simulink model "sim660"  (R2025a)
settings: Solver=ode23s  StartTime=0.0  StopTime=10000  RelTol=1e-3
model workspace (MAT data in the model file):
  op_snapshot1 : opcond.OperatingPoint (value not decoded)
undefined symbols (not defined in the file or in its folder): State132MW, State198MW, State198MW_DELAY
libraries: slpidlib x4, simulink x2, adrc_toolbox_library x1
(part 5 of 5)

== matlab function sim660/Subsystem/MATLAB Function2 ==
  data: pst input; hst input; Dst output; u input
function Dst= Dst(pst,hst,u)
%#codegen

%Dst=u*pst*(-0.0011*hst+4.399);
Dst=0.406*u*pst;
end

== matlab function sim660/MATLAB Function3 ==
  data: Td output; pm input; hm input
function Td = Td(pm, hm)
pm = pm;
hm = hm;
Td = T_ph(pm,hm)-273.15;
end



%% stand alone functions
function T = T_ph(p,h)
% T = T_ph(p,h)
%   Temperature of liquid, vapor or mixture, T [K], as functions of pressure, p [MPa], and enthalpy, h [kJ/kg]
% based on IAPWS-IF97
% Reference: http://www.iapws.org/
% June 2, 2009
% Mark Mikofski
%% size of inputs
dim = size(p);
initnan = NaN(dim);
T = initnan;
%% constants and calculated scalars
Tmin = 273.16; % [K] minimum temperature is triple point
T2bcsat = 554.485; % [K] saturation temperature at 5.85 kJ/kg/K isentropic line between region 2b and 2c
TB13 = 623.15; % [K] temperature at boundary between region 1 and 3
Tmax = 1073.15; % [K] maximum temperature
pmin = psat_T(Tmin); % [MPa] minimum pressure is 611.657 Pa
p2ab = 4; % [MPa] pressure along boundary between region 2a and 2b
p2bcsat = psat_T(T2bcsat); % [MPa] saturation pressure at 5.85 kJ/kg/K isentropic line between region 2b and 2c
pB13sat = psat_T(TB13); % [MPa] saturation pressure at boundary between region 1 and 3, 16.5291643 MPa
pmax = 100; % [MPa] maximum pressure
h1B13L = h1_pT(pB13sat,TB13); % [kJ/kg] saturated liquid enthalpy at boundary between region 1, region 3 and region 4
h2B13V = h2_pT(pB13sat,TB13); % [kJ/kg] saturated vapor enthalpy at boundary between region 2, region 3 and region 4
%% calculated matrices
Tsat = Tsat_p(p); % [K] saturation temperatures
h1min = initnan;h2max = initnan;valid = p>=pmin & p<=pmax;pvalid = p(valid); % initialize matricies with NaN and set valid range of parameters
if any(any(valid))
    Tmin = Tmin*ones(dim);Tmax = Tmax*ones(dim); % copy to matrix of size dim
    h1min(valid) = h1_pT(pvalid,Tmin(valid)); % [kJ/kg] minimum enthalpies
    h2max(valid) = h2_pT(pvalid,Tmax(valid)); % [kJ/kg] maximum enthalpies in region 2
end
h1L = initnan;h2V = initnan;valid = p>=pmin & p<=pB13sat;pvalid = p(valid); % initialize matricies with NaN and set valid range of parameters
if any(any(valid))
    h1L(valid) = h1_pT(pvalid,Tsat(valid)); % [kJ/kg] saturated liquid enthalpies in region 1
    h2V(valid) = h2_pT(pvalid,Tsat(valid)); % [kJ/kg] saturated vapor enthalpies in region 2
end
h1B13 = initnan;h3ab = initnan;h2B23 = initnan;valid = p>=pB13sat & p<=pmax;pvalid = p(valid); % initialize matricies with NaN and set valid range of parameters
if any(any(valid))
    TB13 = TB13*ones(dim); % copy to matrix of size dim
    h1B13(valid) = h1_pT(pvalid,TB13(valid)); % [kJ/kg] enthalpies on boundary between region 1 and region 3
    h3ab(valid) = h3ab_p(pvalid); % [kJ/kg] enthalpies on critical entropy isentropic line between regions 3a and region 3b
    h2B23(valid) = h2_pT(pvalid,TB23_p(pvalid)); % [kJ/kg] enthalpies on boundary between region 2 and region 3
end
h2bc = initnan;valid = p>=p2bcsat & p<=pmax; % initialize matricies with NaN and set valid range of parameters
h2bc(valid) = h2bc_p(p(valid)); % [kJ/kg] enthalpies on boundary between region 2b and 2c
p3sat = pB13sat*ones(dim);valid = h>=h1B13L & h<=h2B13V; % % do NOT use NaN to initialize p3sat, b/c for h<h1B13L or h>h2B13V p>NaN = 0, instead use pB13sat
if any(any(valid))
    p3sat(valid) = p3sat_h(h(valid)); % [MPa] saturation pressure on boundary between region 3 and 4
end
%% valid ranges
valid1 = (p>=pmin & p<=pB13sat & h>=h1min & h<=h1L) | (p>pB13sat & p<=pmax & h>=h1min & h<=h1B13); % valid range for region 1
valid2a = p>=pmin & p<=p2ab & h>h2V & h<=h2max; % valid range for region 2a
valid2b = (p>p2ab & p<=p2bcsat & h>h2V & h<=h2max) | (p>p2bcsat & p<=pmax & h>h2bc & h<=h2max); % valid range for region 2b
valid2c = (p>p2bcsat & p<=pB13sat & h>h2V & h<=h2bc) | (p>pB13sat & p<=pmax & h>h2B23 & h<=h2bc); % valid range for region 2c
valid3a = p>p3sat & p<=pmax & h>h1B13 & h<=h3ab; % valid range for region 3a
valid3b = p>p3sat & p<=pmax & h>h3ab & h<=h2B23; % valid range for region 3b
valid4 = (p>=pmin & p<=pB13sat & h>h1L & h<=h2V) | (p>pB13sat & p<=p3sat & h>h1B13L & h<=h2B13V); % valid range for region 4
if any(any(valid1))
    T(valid1) = T1_ph(p(valid1),h(valid1));
end
if any(any(valid2a))
    T(valid2a) = T2a_ph(p(valid2a),h(valid2a));
end
if any(any(valid2b))
    T(valid2b) = T2b_ph(p(valid2b),h(valid2b));
end
if any(any(valid2c))
    T(valid2c) = T2c_ph(p(valid2c),h(valid2c));
end
if any(any(valid3a))
    T(valid3a) = T3a_ph(p(valid3a),h(valid3a));
end
if any(any(valid3b))
    T(valid3b) = T3b_ph(p(valid3b),h(valid3b));
end
if any(any(valid4))
    T(valid4) = Tsat(valid4);
end
end
function p = psat_T(T)
% p = psat_T(T)
%   Pressure of saturated liquid, mixture or steam, p [MPa], as a function of temperature, T [K]
% based on IAPWS-IF97
% Reference: http://www.iapws.org/
% June 9, 2009
% Mark Mikofski
dim = size(T);
p = NaN(dim);
Tmin = 273.16; % [K] minimum temperature is triple point
Tc = 647.096; % [K] critical point temperature
valid = T>=Tmin & T<=Tc;
pstar = 1; % [Mpa]
Tstar = 1; % [K]
n = [1167.05214527670;-724213.167032060;-17.0738469400920;12020.8247024700;-3232555.03223330;14.9151086135300; ...
    -4823.26573615910;405113.405420570;-0.238555575678490;650.175348447980];
upsilon = T(valid)/Tstar + n(9)./(T(valid)/Tstar-n(10));
A = (upsilon + n(1)).*upsilon + n(2); % use Horner's Method to speed up calculations
B = (n(3)*upsilon + n(4)).*upsilon + n(5); % use Horner's Method to speed up calculations
C = (n(6)*upsilon + n(7)).*upsilon + n(8); % use Horner's Method to speed up calculations
beta = 2*C./(-B + (B.^2 - 4*A.*C).^0.5);
p(valid) = (beta.^4) * pstar;
end
function T = Tsat_p(p)
% T = Tsat_p(p)
%   Temperature of saturated liquid, mixture or steam, T [K], as a function of temperature, p [MPa]
% based on IAPWS-IF97
% Reference: http://www.iapws.org/
% June 9, 2009
% Mark Mikofski
dim = size(p);
T = NaN(dim);
Tmin = 273.16; % [K] minimum temperature is triple point
pmin = psat_T(Tmin); % [MPa] minimum pressure is 611.657 Pa
pc = 22.064; % [MPa] critical pressure
valid = p>=pmin & p<=pc; % initialize matricies with NaN and set valid range of parameters
pstar = 1; % [Mpa]
Tstar = 1; % [K]
n = [1167.05214527670;-724213.167032060;-17.0738469400920;12020.8247024700;-3232555.03223330;14.9151086135300; ...
    -4823.26573615910;405113.405420570;-0.238555575678490;650.175348447980];
beta = (p(valid)/pstar).^0.25;
E = (beta + n(3)).*beta + n(6); % use Horner's Method to speed up calculations
F = (n(1)*beta + n(4)).*beta + n(7); % use Horner's Method to speed up calculations
G = (n(2)*beta + n(5)).*beta + n(8); % use Horner's Method to speed up calculations
D = 2*G./(-F - (F.^2 - 4*E.*G).^0.5);
n11 = n(10) + D;
theta = (n11 - (n11.^2 - 4*(n(9) + n(10)*D)).^0.5)/2;
T(valid) = theta*Tstar;
end
%% basic and fundamental functions
function h = h1_pT(p,T) % [kJ/kg]
R = 0.461526; % [kJ/kg/K] specific gas constant
Tstar = 1386; % [K]
h = R*Tstar*dgammadtau1_pT(p,T);
end
function h = h2_pT(p,T) % [kJ/kg]
R = 0.461526; % [kJ/kg/K] specific gas constant
Tstar = 540; % [K]
h = R*Tstar*dgammadtau2_pT(p,T);
end
function dgammadtau = dgammadtau1_pT(p,T)
dim = length(p);
pstar = 16.53; % [MPa]
Tstar = 1386; % [K]
pi = p/pstar;
tau = Tstar./T;
I = [0,0,0,0,0,0,0,0,1,1,1,1,1,1,2,2,2,2,2,3,3,3,4,4,4,5,8,8,21,23,29,30,31,32];
J = [-2,-1,0,1,2,3,4,5,-9,-7,-1,0,1,3,-3,0,1,3,17,-4,0,6,-5,-2,10,-8,-11,-6,-29,-31,-38,-39,-40,-41];
n = [0.146329712131670,-0.845481871691140,-3.75636036720400,3.38551691683850,-0.957919633878720,0.157720385132280, ...
    -0.0166164171995010,0.000812146299835680,0.000283190801238040,-0.000607063015658740,-0.0189900682184190, ...
    -0.0325297487705050,-0.0218417171754140,-5.28383579699300e-05,-0.000471843210732670,-0.000300017807930260, ...
    4.76613939069870e-05,-4.41418453308460e-06,-7.26949962975940e-16,-3.16796448450540e-05,-2.82707979853120e-06, ...
    -8.52051281201030e-10,-2.24252819080000e-06,-6.51712228956010e-07,-1.43417299379240e-13,-4.05169968601170e-07, ...
    -1.27343017416410e-09,-1.74248712306340e-10,-6.87621312955310e-19,1.44783078285210e-20,2.63357816627950e-23, ...
    -1.19476226400710e-23,1.82280945814040e-24,-9.35370872924580e-26];
Nterms = 34;
I = ones(dim,1)*I;
J = ones(dim,1)*J;
n = ones(dim,1)*n;
pi = pi*ones(1,Nterms);
tau = tau*ones(1,Nterms);
dgammadtau = sum(n.*(7.1-pi).^I.*J.*(tau-1.222).^(J-1),2);
end
function dgammadtau = dgammadtau2_pT(p,T)
dim = length(p);
pstar = 1; % [MPa] scaling pressure for nondimensional pressure, pi
Tstar = 540; % [K] scaling temperature for nondimensional temperature substitution variable
pi = p/pstar; % nondimensional pressure
tau = Tstar./T; % temperature substitution variable
%% ideal part
J0 = [0,1,-5,-4,-3,-2,-1,2,3]; % ideal part exponenets
n0 = [-9.69276865002170,10.0866559680180,-0.00560879112830200,0.0714527380814550,-0.407104982239280,1.42408191714440, ...
    -4.38395113194500,-0.284086324607720,0.0212684637533070];
N0terms = 9; % number of ideal terms in summation
J0 = ones(dim,1)*J0;
n0 = ones(dim,1)*n0;
tau0 = tau*ones(1,N0terms);
dgammadtau0 = sum(n0.*J0.*tau0.^(J0-1),2); % index sums of valid inputs into corresponding location in output array
%% residual part
IR = [1,1,1,1,1,2,2,2,2,2,3,3,3,3,3,4,4,4,5,6,6,6,7,7,7,8,8,9,10,10,10,16,16,18,20,20,20,21,22,23,24,24,24];
JR = [0,1,2,3,6,1,2,4,7,36,0,1,3,6,35,1,2,3,7,3,16,35,0,11,25,8,36,13,4,10,14,29,50,57,20,35,48,21,53,39,26,40,58];
nR = [-0.00177317424732130,-0.0178348622923580,-0.0459960136963650,-0.0575812590834320,-0.0503252787279300, ...
    -3.30326416702030e-05,-0.000189489875163150,-0.00393927772433550,-0.0437972956505730,-2.66745479140870e-05, ...
    2.04817376923090e-08,4.38706672844350e-07,-3.22776772385700e-05,-0.00150339245421480,-0.0406682535626490, ...
    -7.88473095593670e-10,1.27907178522850e-08,4.82253727185070e-07,2.29220763376610e-06,-1.67147664510610e-11, ...
    -0.00211714723213550,-23.8957419341040,-5.90595643242700e-18,-1.26218088991010e-06,-0.0389468424357390, ...
    1.12562113604590e-11,-8.23113408979980,1.98097128020880e-08,1.04069652101740e-19,-1.02347470959290e-13, ...
    -1.00181793795110e-09,-8.08829086469850e-11,0.106930318794090,-0.336622505741710,8.91858453554210e-25, ...
    3.06293168762320e-13,-4.20024676982080e-06,-5.90560296856390e-26,3.78269476134570e-06,-1.27686089346810e-15, ...
    7.30876105950610e-29,5.54147153507780e-17,-9.43697072412100e-07];
NRterms = 43;
IR = ones(dim,1)*IR;
JR = ones(dim,1)*JR;
nR = ones(dim,1)*nR;
pi = pi*ones(1,NRterms);
tauR = tau*ones(1,NRterms);
dgammadtauR = sum(nR.*pi.^IR.*JR.*(tauR-0.5).^(JR-1),2);
dgammadtau = dgammadtau0 + dgammadtauR;
end
function T = T1_ph(p,h) % [K]
dim = length(p);
pstar = 1; % [MPa]
Tstar = 1; % [K]
hstar = 2500; % [kJ/kg]
pi = p/pstar;
eta = h/hstar;
I = [0,0,0,0,0,0,1,1,1,1,1,1,1,2,2,3,3,4,5,6];
J = [0,1,2,6,22,32,0,1,2,3,4,10,32,10,32,10,32,32,32,32];
n = [-238.724899245210,404.211886379450,113.497468817180,-5.84576160480390,-0.000152854824131400,-1.08667076953770e-06, ...
    -13.3917448726020,43.2110391835590,-54.0100671705060,30.5358922039160,-6.59647494236380,0.00939654008783630, ...
    1.15736475053400e-07,-2.58586412820730e-05,-4.06443630847990e-09,6.64561861916350e-08,8.06707341030270e-11, ...
    -9.34777712139470e-13,5.82654420206010e-15,-1.50201859535030e-17];
Nterms = 20;
I = ones(dim,1)*I;
J = ones(dim,1)*J;
n = ones(dim,1)*n;
pi = pi*ones(1,Nterms);
eta = eta*ones(1,Nterms);
theta = sum(n.*pi.^I.*(eta+1).^J,2);
T = Tstar*theta;
end
function T = T2a_ph(p,h) % [K]
dim = length(p);
pstar = 1; % [MPa]
Tstar = 1; % [K]
hstar = 2000; % [kJ/kg]
pi = p/pstar;
eta = h/hstar;
Ia = [0,0,0,0,0,0,1,1,1,1,1,1,1,1,1,2,2,2,2,2,2,2,2,3,3,4,4,4,5,5,5,6,6,7];
Ja = [0,1,2,3,7,20,0,1,2,3,7,9,11,18,44,0,2,7,36,38,40,42,44,24,44,12,32,44,32,36,42,34,44,28];
na = [1089.89523182880,849.516544955350,-107.817480918260,33.1536548012630,-7.42320167902480,11.7650487243560, ...
    1.84457493557900,-4.17927005496240,6.24781969358120,-17.3445631081140,-200.581768620960,271.960654737960, ...
    -455.113182858180,3091.96886047550,252266.403578720,-0.00617074228683390,-0.310780466295830,11.6708730771070, ...
    128127984.040460,-985549096.232760,2822454697.30020,-3594897141.07030,1722734991.31970,-13551.3342407750, ...
    12848734.6646500,1.38657242832260,235988.325565140,-13105236.5450540,7399.98354747660,-551966.970300600, ...
    3715408.59962330,19127.7292396600,-415351.648356340,-62.4598551925070];
Naterms = 34;
Ia = ones(dim,1)*Ia;
Ja = ones(dim,1)*Ja;
na = ones(dim,1)*na;
pi = pi*ones(1,Naterms);
eta = eta*ones(1,Naterms);
theta = sum(na.*pi.^Ia.*(eta-2.1).^Ja,2);
T = Tstar*theta;
end
function T = T2b_ph(p,h) % [K]
dim = length(p);
pstar = 1; % [MPa]
Tstar = 1; % [K]
hstar = 2000; % [kJ/kg]
pi = p/pstar;
eta = h/hstar;
Ib = [0,0,0,0,0,0,0,0,1,1,1,1,1,1,1,1,2,2,2,2,3,3,3,3,4,4,4,4,4,4,5,5,5,6,7,7,9,9];
Jb = [0,1,2,12,18,24,28,40,0,2,6,12,18,24,28,40,2,8,18,40,1,2,12,24,2,12,18,24,28,40,18,24,40,28,2,28,1,40];
nb = [1489.50410795160,743.077983140340,-97.7083187978370,2.47424647056740,-0.632813200160260,1.13859521296580, ...
    -0.478118636486250,0.00852081234315440,0.937471473779320,3.35931186049160,3.38093556014540,0.168445396719040, ...
    0.738757452366950,-0.471287374361860,0.150202731397070,-0.00217641142197500,-0.0218107553247610,-0.108297844036770, ...
    -0.0463333246358120,7.12803519595510e-05,0.000110328317899990,0.000189552483879020,0.00308915411605370, ...
    0.00135555045549490,2.86402374774560e-07,-1.07798573575120e-05,-7.64627124548140e-05,1.40523928183160e-05, ...
    -3.10838143314340e-05,-1.03027382121030e-06,2.82172816350400e-07,1.27049022719450e-06,7.38033534682920e-08, ...
    -1.10301392389090e-08,-8.14563652078330e-14,-2.51805456829620e-11,-1.75652339694070e-18,8.69341563441630e-15];
Nbterms = 38;
Ib = ones(dim,1)*Ib;
Jb = ones(dim,1)*Jb;
nb = ones(dim,1)*nb;
pi = pi*ones(1,Nbterms);
eta = eta*ones(1,Nbterms);
theta = sum(nb.*(pi-2).^Ib.*(eta-2.6).^Jb,2);
T = Tstar*theta;
end
function T = T2c_ph(p,h) % [K]
dim = length(p);
pstar = 1; % [MPa]
Tstar = 1; % [K]
hstar = 2000; % [kJ/kg]
pi = p/pstar;
eta = h/hstar;
Ic = [-7,-7,-6,-6,-5,-5,-2,-2,-1,-1,0,0,1,1,2,6,6,6,6,6,6,6,6];
Jc = [0,4,0,2,0,2,0,1,0,2,0,1,4,8,4,0,1,4,10,12,16,20,22];
nc = [-3236839855524.20,7326335090218.10,358250899454.470,-583401318515.900,-10783068217.4700,20825544563.1710, ...
    610747.835645160,859777.225355800,-25745.7236041700,31081.0884227140,1208.23158659360,482.197551092550, ...
    3.79660012724860,-10.8429848800770,-0.0453641726766600,1.45591156586980e-13,1.12615974072300e-12,-1.78049822406860e-11, ...
    1.23245796908320e-07,-1.16069211309840e-06,2.78463670885540e-05,-0.000592700384741760,0.00129185829918780];
Ncterms = 23;
Ic = ones(dim,1)*Ic;
Jc = ones(dim,1)*Jc;
nc = ones(dim,1)*nc;
pi = pi*ones(1,Ncterms);
eta = eta*ones(1,Ncterms);
theta = sum(nc.*(pi+25).^Ic.*(eta-1.8).^Jc,2);
T = Tstar*theta;
end
function T = T3a_ph(p,h) % [K]
dim = length(p);
pstar = 100; % [MPa]
Tstar = 760; % [K]
hstar = 2300; % [kJ/kg]
pi = p/pstar;
eta = h/hstar;
I = [-12,-12,-12,-12,-12,-12,-12,-12,-10,-10,-10,-8,-8,-8,-8,-5,-3,-2,-2,-2,-1,-1,0,0,1,3,3,4,4,10,12];
J = [0,1,2,6,14,16,20,22,1,5,12,0,2,4,10,2,0,1,3,4,0,2,0,1,1,0,1,0,3,4,5];
n = [-1.33645667811215e-07,4.55912656802978e-06,-1.46294640700979e-05,0.00639341312970080,372.783927268847, ...
    -7186.54377460447,573494.752103400,-2675693.29111439,-3.34066283302614e-05,-0.0245479214069597,47.8087847764996, ...
    7.64664131818904e-06,0.00128350627676972,0.0171219081377331,-8.51007304583213,-0.0136513461629781, ...
    -3.84460997596657e-06,0.00337423807911655,-0.551624873066791,0.729202277107470,-0.00992522757376041, ...
    -0.119308831407288,0.793929190615421,0.454270731799386,0.209998591259910,-0.00642109823904738,-0.0235155868604540, ...
    0.00252233108341612,-0.00764885133368119,0.0136176427574291,-0.0133027883575669];
Nterms = 31;
I = ones(dim,1)*I;
J = ones(dim,1)*J;
n = ones(dim,1)*n;
pi = pi*ones(1,Nterms);
eta = eta*ones(1,Nterms);
theta = sum(n.*(pi+0.240).^I.*(eta-0.615).^J,2);
T = Tstar*theta;
end
function T = T3b_ph(p,h) % [K]
dim = length(p);
pstar = 100; % [MPa]
Tstar = 860; % [K]
hstar = 2800; % [kJ/kg]
pi = p/pstar;
eta = h/hstar;
I = [-12,-12,-10,-10,-10,-10,-10,-8,-8,-8,-8,-8,-6,-6,-6,-4,-4,-3,-2,-2,-1,-1,-1,-1,-1,-1,0,0,1,3,5,6,8];
J = [0,1,0,1,5,10,12,0,1,2,4,10,0,1,2,0,1,5,0,4,2,4,6,10,14,16,0,2,1,1,1,1,1];
n = [3.23254573644920e-05,-0.000127575556587181,-0.000475851877356068,0.00156183014181602,0.105724860113781, ...
    -85.8514221132534,724.140095480911,0.00296475810273257,-0.00592721983365988,-0.0126305422818666,-0.115716196364853, ...
    84.9000969739595,-0.0108602260086615,0.0154304475328851,0.0750455441524466,0.0252520973612982,-0.0602507901232996, ...
    -3.07622221350501,-0.0574011959864879,5.03471360939849,-0.925081888584834,3.91733882917546,-77.3146007130190, ...
    9493.08762098587,-1410437.19679409,8491662.30819026,0.861095729446704,0.323346442811720,0.873281936020439, ...
    -0.436653048526683,0.286596714529479,-0.131778331276228,0.00676682064330275];
Nterms = 33;
I = ones(dim,1)*I;
J = ones(dim,1)*J;
n = ones(dim,1)*n;
pi = pi*ones(1,Nterms);
eta = eta*ones(1,Nterms);
theta = sum(n.*(pi+0.298).^I.*(eta-0.720).^J,2);
T = Tstar*theta;
end
function h = h2bc_p(p)
pstar = 1; % [MPa]
hstar = 1; % [kJ/kg]
pi = p/pstar;
n = [0.90584278514723e3;-0.67955786399241;0.12809002730136e-3;0.26526571908428e4;0.45257578905948e1];
eta = n(4) + ((pi-n(5))/n(3)).^0.5;
h = eta*hstar;
end
function h = h3ab_p(p)
pstar = 1; % [MPa]
hstar = 1; % [kJ/kg]
pi = p/pstar;
n = [0.201464004206875e4;0.374696550136983e1;-0.219921901054187e-1;0.875131686009950e-4];
eta = n(1) + pi.*(n(2) + pi.*(n(3) + pi*n(4))); % use Horner's Method to speed up calculations
h = eta*hstar;
end
function T = TB23_p(p)
pstar = 1; % [MPa]
Tstar = 1; % [K]
pi = p/pstar;
n = [0.34805185628969e3; -0.11671859879975e1; 0.10192970039326e-2; 0.57254459862746e3; 0.13918839778870e2];
theta = n(4) + ((pi-n(5))/n(3)).^0.5;
T = theta*Tstar;
end
function p = p3sat_h(h)
dim = length(h);
pstar = 22; % [MPa]
hstar = 2600; % [kJ/kg]
eta = h/hstar;
I = [0,1,1,1,1,5,7,8,14,20,22,24,28,36];
J = [0,1,3,4,36,3,0,24,16,16,3,18,8,24];
n = [0.600073641753024,-9.36203654849857,24.6590798594147,-107.014222858224,-91582131580576.8,-8623.32011700662, ...
    -23.5837344740032,2.52304969384128e+17,-3.89718771997719e+18,-3.33775713645296e+22,35649946963.6328, ...
    -1.48547544720641e+26,3.30611514838798e+18,8.13641294467829e+37];
Nterms = 14;
I = ones(dim,1)*I;
J = ones(dim,1)*J;
n = ones(dim,1)*n;
eta = eta*ones(1,Nterms);
pi = sum(n.*(eta-1.02).^I.*(eta-0.608).^J,2);
p = pstar*pi;
end
